simulink model "Astrolab_jumeaunumerique_2015b_v19"  (R2019b)
settings: Solver=FixedStepAuto  StartTime=0.0  StopTime=5  RelTol=1e-3
model workspace (MAT data in the model file):
  Freq = Simulink.Parameter
  Freq.DataType = 'auto'
  Freq.DocUnits = 'Hz'
  Freq.Dimensions = [0 0]
libraries: eePwmGenerator x2
settings Model: Creator=utilisateur  LastModifiedBy=Pr Goedz 974
settings RTWCC: Description=Generic Real-Time Target

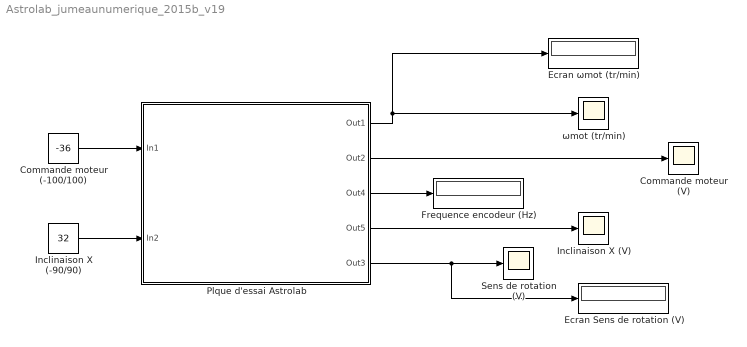
== system Astrolab_jumeaunumerique_2015b_v19 ==
  Commande moteur (-100/100) : Constant  Value=-36
  Commande moteur (V) : Scope
  Ecran Sens de rotation (V) : Display
  Ecran ωmot (tr/min) : Display
  Frequence encodeur (Hz) : Display
  Inclinaison X (-90/90) : Constant  Value=32
  Inclinaison X (V) : Scope
  Plque d'essai Astrolab : Subsystem
      mask Display: image('$imagefile'); % Use "Edit Image" on toolstrip to change.
  Sens de rotation (V) : Scope
  ωmot (tr/min) : Scope
  wires:
  Plque d'essai Astrolab/1(Out1) -> Ecran ωmot (tr/min)/1, ωmot (tr/min)/1
  Plque d'essai Astrolab/2(Out2) -> Commande moteur (V)/1
  Plque d'essai Astrolab/3(Out4) -> Frequence encodeur (Hz)/1
  Plque d'essai Astrolab/4(Out5) -> Inclinaison X (V)/1
  Inclinaison X (-90/90)/1 -> Plque d'essai Astrolab/2(In2)
  Commande moteur (-100/100)/1 -> Plque d'essai Astrolab/1(In1)
  Plque d'essai Astrolab/5(Out3) -> Ecran Sens de rotation (V)/1, Sens de rotation (V)/1

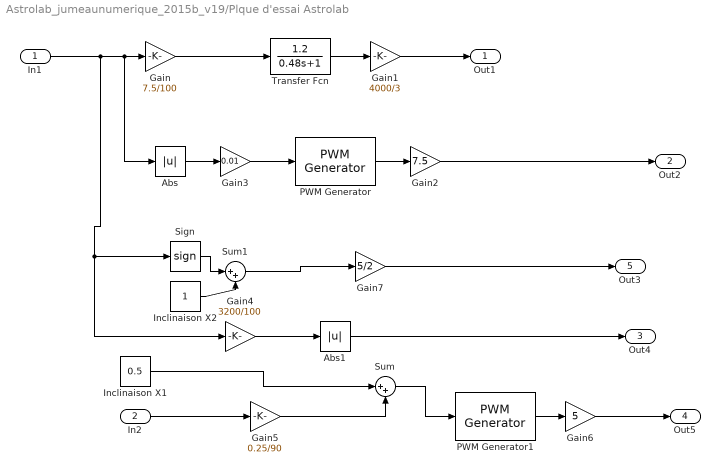
== system Astrolab_jumeaunumerique_2015b_v19/Plque d'essai Astrolab ==
  In1 : Inport
  In2 : Inport  Port=2
  Abs : Abs
  Abs1 : Abs
  Gain : Gain  Gain=7.5/100
  Gain1 : Gain  Gain=4000/3
  Gain2 : Gain  Gain=7.5
  Gain3 : Gain  Gain=0.01
  Gain4 : Gain  Gain=3200/100
  Gain5 : Gain  Gain=0.25/90
  Gain6 : Gain  Gain=5
  Gain7 : Gain  Gain=5/2
  Inclinaison X1 : Constant  Value=0.5
  Inclinaison X2 : Constant
  PWM Generator : eePwmGenerator/PWM Generator  CarrCount=Up  Tper=0.001  Ts=5e-5
  PWM Generator1 : eePwmGenerator/PWM Generator  CarrCount=Up  Tper=0.001  Ts=5e-5
  Sign : Signum
  Sum : Sum  Inputs=|++
  Sum1 : Sum  Inputs=|++
  Transfer Fcn : TransferFcn  Numerator=[1.2]  Denominator=[0.48 1]
  Out1 : Outport
  Out2 : Outport  Port=2
  Out4 : Outport  Port=3
  Out5 : Outport  Port=4
  Out3 : Outport  Port=5
  wires:
  PWM Generator/1 -> Gain2/1
  In1/1 -> Sign/1, Gain4/1, Abs/1, Gain/1
  Gain2/1 -> Out2/1
  Gain3/1 -> PWM Generator/1
  Transfer Fcn/1 -> Gain1/1
  Sum/1 -> PWM Generator1/1
  PWM Generator1/1 -> Gain6/1
  Gain/1 -> Transfer Fcn/1
  In2/1 -> Gain5/1
  Inclinaison X1/1 -> Sum/1
  Gain5/1 -> Sum/2
  Gain1/1 -> Out1/1
  Gain4/1 -> Abs1/1
  Gain6/1 -> Out5/1
  Sum1/1 -> Gain7/1
  Sign/1 -> Sum1/1
  Gain7/1 -> Out3/1
  Inclinaison X2/1 -> Sum1/2
  Abs/1 -> Gain3/1
  Abs1/1 -> Out4/1
